simulink model "Encoding_Unstable_system"  (R2021a)
settings: Solver=VariableStepAuto  StartTime=0.0  StopTime=100  RelTol=1e-3
values from neighbouring files (symbols this model uses):
  sample_time = 1    [main1.m]    (also in main2.m)
undefined symbols (not defined in the file or in its folder): Discrete, Time
libraries: dspsrcs4 x2, ctrlSharedLib x1
settings Model: Creator=mehra  LastModifiedBy=mehra

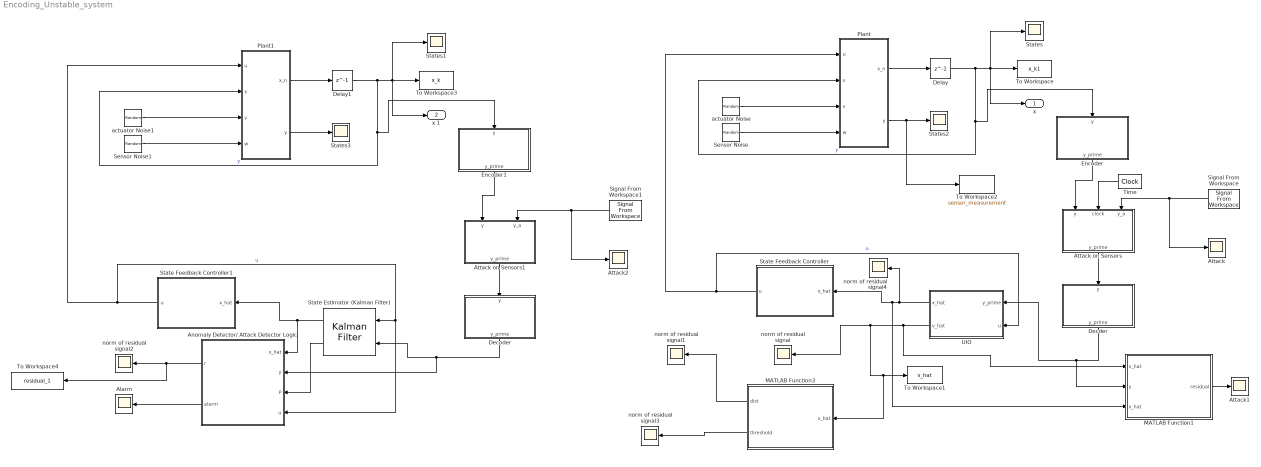
== system Encoding_Unstable_system ==
  Alarm : Scope
  Anomaly Detector/ Attack Detector Logic : MATLAB Function  TreatAsAtomicUnit=on
  Attack : Scope
  Attack on Sensors : MATLAB Function  TreatAsAtomicUnit=on
  Attack on Sensors1 : MATLAB Function  TreatAsAtomicUnit=on
  Attack1 : Scope
  Attack2 : Scope
  Decder : MATLAB Function  TreatAsAtomicUnit=on
  Decoder : MATLAB Function  TreatAsAtomicUnit=on
  Delay : Delay  DelayLength=1  InitialCondition=[0;0]  SampleTime=sample_time
  Delay1 : Delay  DelayLength=1  InitialCondition=[0;0]  SampleTime=sample_time
  Encoder : MATLAB Function  TreatAsAtomicUnit=on
  Encoder1 : MATLAB Function  TreatAsAtomicUnit=on
  MATLAB Function1 : MATLAB Function  TreatAsAtomicUnit=on
  MATLAB Function3 : MATLAB Function  TreatAsAtomicUnit=on
  Plant : MATLAB Function  TreatAsAtomicUnit=on
  Plant1 : MATLAB Function  TreatAsAtomicUnit=on
  Sensor Noise : RandomNumber  Mean=[0 0]  Variance=[0.0001 0.0001]  Seed=[randi(100) randi(100)]  SampleTime=sample_time
  Sensor Noise1 : RandomNumber  Mean=[0 0]  Variance=[0.01 0.01]  Seed=[randi(100) randi(100)]  SampleTime=sample_time
  Signal From Workspace : dspsrcs4/Signal From Workspace  X=y_a  Ts=sample_time  nsamps=1  OutputAfterFinalValue=Cyclic repetition  ignoreOrWarnInputAndFrameLengths=off  OutputFrames=off
  Signal From Workspace1 : dspsrcs4/Signal From Workspace  X=y_a  Ts=sample_time  nsamps=1  OutputAfterFinalValue=Cyclic repetition  ignoreOrWarnInputAndFrameLengths=off  OutputFrames=off
  State Estimator (Kalman Filter) : ctrlSharedLib/Kalman Filter  TimeDomain=Discrete-Time  UseCurrentEstimator=on  ModelSource=Individual A, B, C, D matrices  ModelSourceVariable=ss(0.95,1,1,0,1)  A=[0.8 0; 0.5 1]  B=[1;0.5]  C=[2 0.5;0 1]  D=0  NumberOfStates=1  NumberOfInputs=1  NumberOfOutputs=1  InitialEstimateSource=Dialog  X0=[0 0]'  P0=10  UseK=off  UseGH=off  NumberOfProcessNoiseInputs=1  G=1  TimeInvariantG=on  H=0  TimeInvariantH=on  Q=0.001  TimeInvariantQ=on  R=0.001  TimeInvariantR=on  N=0  TimeInvariantN=on  AddInputPort=on  AddEnablePort=off  OutputEstimatedY=off  OutputP=on  Ts=sample_time
  State Feedback Controller : MATLAB Function  TreatAsAtomicUnit=on
  State Feedback Controller1 : MATLAB Function  TreatAsAtomicUnit=on
  States{,1..3} (4 alike) : Scope
  Time : DigitalClock  SampleTime=sample_time
  To Workspace : ToWorkspace  VariableName=x_k1  SaveFormat=Timeseries  SampleTime=sample_time
  To Workspace1 : ToWorkspace  VariableName=v_hat  SaveFormat=Timeseries  SampleTime=sample_time
  To Workspace2 : ToWorkspace  VariableName=sensor_measurement  SaveFormat=Timeseries  SampleTime=sample_time
  To Workspace3 : ToWorkspace  VariableName=x_k  SaveFormat=Timeseries  SampleTime=sample_time
  To Workspace4 : ToWorkspace  VariableName=residual_1  SaveFormat=Timeseries  SampleTime=sample_time
  UIO : Subsystem
  actuator Noise : RandomNumber  Mean=[0 0]  Variance=[0.0001 0.0001]  Seed=[randi(100) randi(100)]  SampleTime=sample_time
  actuator Noise1 : RandomNumber  Mean=[0 0]  Variance=[0.0001 0.0001]  Seed=[randi(100) randi(100)]  SampleTime=sample_time
  norm of residual signal{,1..4} (5 alike) : Scope
  "x " : Outport  VectorParamsAs1DForOutWhenUnconnected=off
  x 1 : Outport  Port=2  VectorParamsAs1DForOutWhenUnconnected=off
  wires:
  Time/1 -> Attack on Sensors/2(clock)
  Signal From Workspace/1 -> Attack/1, Attack on Sensors/3(y_a)
  Encoder/1(y_prime) -> Attack on Sensors/1(y)
  Plant/2(y) -> To Workspace2/1, States2/1
  Decder/1(y_prime) -> MATLAB Function1/2(y), UIO/1(y_prime)
  actuator Noise/1 -> Plant/3(v)
  State Feedback Controller/1(u) -> UIO/2(u), Plant/1(u)  "u"
  Delay/1 -> "x "/1, States/1, To Workspace/1, Plant/2(x), Encoder/1(y)  "y"
  Attack on Sensors/1(y_prime) -> Decder/1(y)
  Sensor Noise/1 -> Plant/4(w)
  Plant/1(x_n) -> Delay/1
  UIO/1(x_hat) -> norm of residual signal4/1, MATLAB Function1/3(x_hat), State Feedback Controller/1(x_hat)
  UIO/2(v_hat) -> MATLAB Function1/1(v_hat), MATLAB Function3/1(v_hat), To Workspace1/1, norm of residual signal/1
  MATLAB Function3/1(dist) -> norm of residual signal1/1
  MATLAB Function3/2(threshold) -> norm of residual signal3/1
  MATLAB Function1/1(residual) -> Attack1/1
  State Estimator (Kalman Filter)/2 -> Anomaly Detector/ Attack Detector Logic/3(P)
  State Feedback Controller1/1(u) -> State Estimator (Kalman Filter)/1, Anomaly Detector/ Attack Detector Logic/4(u), Plant1/1(u)  "u"
  Anomaly Detector/ Attack Detector Logic/2(alarm) -> Alarm/1
  actuator Noise1/1 -> Plant1/3(v)
  Decoder/1(y_prime) -> Anomaly Detector/ Attack Detector Logic/2(y), State Estimator (Kalman Filter)/2
  Signal From Workspace1/1 -> Attack2/1, Attack on Sensors1/2(y_a)
  Anomaly Detector/ Attack Detector Logic/1(r) -> To Workspace4/1, norm of residual signal2/1
  Attack on Sensors1/1(y_prime) -> Decoder/1(y)
  Encoder1/1(y_prime) -> Attack on Sensors1/1(y)
  Delay1/1 -> x 1/1, States1/1, To Workspace3/1, Plant1/2(x), Encoder1/1(y)  "y"
  Plant1/2(y) -> States3/1
  State Estimator (Kalman Filter)/1 -> Anomaly Detector/ Attack Detector Logic/1(x_hat), State Feedback Controller1/1(x_hat)
  Sensor Noise1/1 -> Plant1/4(w)
  Plant1/1(x_n) -> Delay1/1

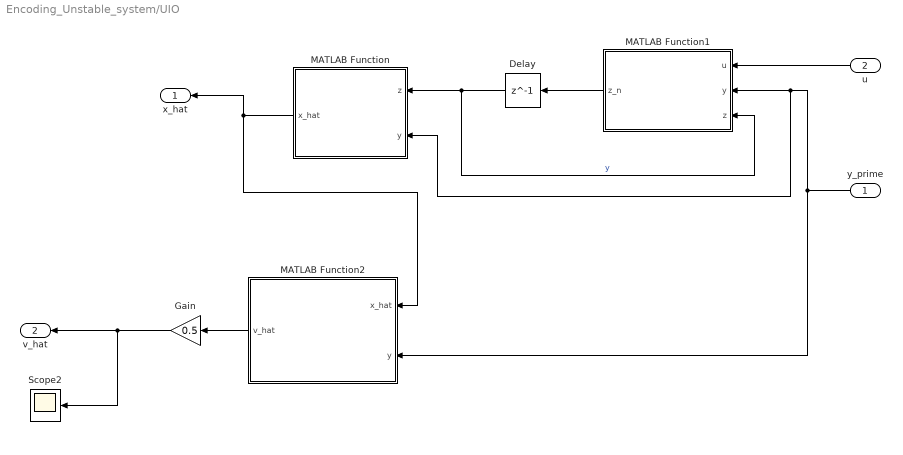
== system Encoding_Unstable_system/UIO ==
  y_prime : Inport
  u : Inport  Port=2
  Delay : Delay  DelayLength=1  InitialCondition=zeros(2,1)
  Gain : Gain  Gain=0.5
  MATLAB Function : MATLAB Function  TreatAsAtomicUnit=on
  MATLAB Function1 : MATLAB Function  TreatAsAtomicUnit=on
  MATLAB Function2 : MATLAB Function  TreatAsAtomicUnit=on
  Scope2 : Scope
  x_hat : Outport  VectorParamsAs1DForOutWhenUnconnected=off
  v_hat : Outport  Port=2  VectorParamsAs1DForOutWhenUnconnected=off
  wires:
  MATLAB Function1/1(z_n) -> Delay/1
  u/1 -> MATLAB Function1/1(u)
  y_prime/1 -> MATLAB Function/2(y), MATLAB Function1/2(y), MATLAB Function2/2(y)
  Delay/1 -> MATLAB Function1/3(z), MATLAB Function/1(z)  "y"
  MATLAB Function/1(x_hat) -> x_hat/1, MATLAB Function2/1(x_hat)
  MATLAB Function2/1(v_hat) -> Gain/1
  Gain/1 -> Scope2/1, v_hat/1

== matlab function Encoding_Unstable_system/Anomaly Detector// Attack Detector Logic ==
  data: x_hat input; y input; r output; P input; alarm output; u input
function [r, alarm] = Detector(x_hat,y, P, u)
% this function should contain the detection strategy

% for the chi square detector "P" should be the name of detection signal and
% "tau" the name of threshold
A = [0.8 0; 0.5 1];
B = [1;0.5];
C = [2 0.5;0 1];
threshold = chi2inv(0.99,2);
sigma = ((C)*(P)*(C')) + 0.01;
r = 0.8*norm(y' - C*(A*x_hat + B*u),2);
z = (r') * (inv(sigma)) * r;
if z<=threshold
    alarm = 0;
else
    alarm = 1;
end
alarm = alarm;
residual = z;
threshold = threshold;
end

== matlab function Encoding_Unstable_system/Attack on Sensors1 ==
  data: y input; y_prime output; y_a input
function y_prime = fcn(y, y_a)
% this function should contain the attacker action on the sensor
% measurements
sigma1 = [2 -0.5;-0.5 1];
sigma2 = [1 -1;2 0];

y_prime = y_a;
% y_prime = y;

end

== matlab function Encoding_Unstable_system/Decoder ==
  data: y input; y_prime output
function y_prime = fcn(y)
% this function should contain the attacker action on the sensor
% measurements
sigma1 = [2 -0.5;-0.5 1];
sigma2 = [1 -1;2 0];
% y_prime = y*inv(sigma1);
y_prime = y;
end

== matlab function Encoding_Unstable_system/Encoder1 ==
  data: y input; y_prime output
function y_prime = fcn(y)
% this function should contain the attacker action on the sensor
% measurements
sigma1 = [2 -0.5;-0.5 1];
sigma2 = [1 -1;2 0];
% y_prime = y'*sigma1;
y_prime = y;
end

== matlab function Encoding_Unstable_system/Plant1 ==
  data: x_n output; u input; y output; x input; v input; w input
function [x_n, y] = fcn(u, x, v, w)

%A=[1.0000    0.0001   -0.0010;0.5747    1.0000   -0.0003;0.0162    0.0000    1.0000];
%B = [0.1   -0.2; -0.0536    0.0332;0.1955   -0.5294];

A = [0.8 0; 0.5 1];
B = [1;0.5];
C = [2 0.5;0 1];
D = 0;

x_n = A*x + B*u + v;
y = C*x + D*u + w;

== matlab function Encoding_Unstable_system/State Feedback Controller1 ==
  data: x_hat input; u output
function u  = Controller(x_hat)
%two tanks model 



K = [-1  -4];

u = K*x_hat;

== matlab function Encoding_Unstable_system/Plant ==
  data: x_n output; u input; y output; x input; v input; w input
function [x_n, y] = fcn(u, x, v, w)

%A=[1.0000    0.0001   -0.0010;0.5747    1.0000   -0.0003;0.0162    0.0000    1.0000];
%B = [0.1   -0.2; -0.0536    0.0332;0.1955   -0.5294];

A = [0.8 0; 0.5 1];
B = [1;0.5];
C = [2 0.5;0 1];
D = 0;

x_n = A*x + B*u + v;
y = C*x + D*u + w;

== matlab function Encoding_Unstable_system/Attack on Sensors ==
  data: y input; y_prime output; clock input; y_a input
function y_prime = fcn(y, clock, y_a)
% this function should contain the attacker action on the sensor
% measurements
sigma1 = [2 -0.5;-0.5 1];
sigma2 = [1 -1;2 0];

% y_prime = y_a;
y_prime = y;

end

== matlab function Encoding_Unstable_system/State Feedback Controller ==
  data: x_hat input; u output
function u  = Controller(x_hat)
%two tanks model 



K = [0.1 -0.1];

u = K*x_hat;

== matlab function Encoding_Unstable_system/MATLAB Function3 ==
  data: v_hat input; dist output; threshold output
function [dist,threshold] = Anomaly_Detector(v_hat)


sigma = 0.0136;
mu = 0;
% a = 0.0150;
% b = sqrt(2*pi);
% c = 1/(a.*b);
c = sqrt(sigma) * sqrt(2*pi)
% dist = (1./c) *(exp(-0.5*(1/sigma)*(v_hat - mu)^2))*1/29.5893;
dist = abs(log2(1/(2*pi*sigma)*exp(-(v_hat-mu).^2/(2*sigma^2)))/2.5);


% pd = makedist('Normal','mu',mu,'sigma',sigma);
% dist = pdf(pd,v_hat)
threshold = 0.9;

if dist<threshold
    alarm = 1;
%     prob = 0;
% abs(v_hat) <= 0.13
else
    alarm = 0;
%     prob = 1;



end

== matlab function Encoding_Unstable_system/Encoder ==
  data: y input; y_prime output
function y_prime = fcn(y)
% this function should contain the attacker action on the sensor
% measurements

trans = [-0.547381274157748,0.836883349518582;0.836883349518582,0.547381274157748];

y_prime = y'*trans;
% y_prime = y;
end

== matlab function Encoding_Unstable_system/Decder ==
  data: y input; y_prime output
function y_prime = fcn(y)
% this function should contain the attacker action on the sensor
% measurements
trans = [-0.547381274157748,0.836883349518582;0.836883349518582,0.547381274157748];

y_prime = y*trans';
% y_prime = y;
end

== matlab function Encoding_Unstable_system/UIO/MATLAB Function ==
  data: z input; x_hat output; y input
function x_hat = estimator(z,y)

M = [0.666666666666667,-0.666666666666667;
    0.666666666666667,-0.666666666666667];

x_hat = z + M*y';

== matlab function Encoding_Unstable_system/UIO/MATLAB Function1 ==
  data: u input; z_n output; y input; z input
function z_n = UIO(u,y,z)

A = [0.8 0; 0.5 1];
B = [1;0.5];
C = [2 0.5;0 1];
D = 0;

M = [0.666666666666667,-0.666666666666667;
    0.666666666666667,-0.666666666666667];




L6 = [-0.0515    0.3474;
   -0.2058    1.3897];

z_n = (eye(2)-M*C)*(A*z + A*M*y'+B*u) + L6*(y' - C*z - C*M*y');

x_hat = z + M*y';

== matlab function Encoding_Unstable_system/UIO/MATLAB Function2 ==
  data: x_hat input; v_hat output; y input
function v_hat = unknown_estimator(x_hat,y)

A = [0.8 0; 0.5 1];
B = [1;0.5];
C = [2 0.5;0 1];
% D = 0;

E = [1;1];
D = [1;1];

v_hat = pinv(D)*y' - pinv(D)*C*x_hat;

== matlab function Encoding_Unstable_system/MATLAB Function1 ==
  data: v_hat input; residual output; y input; x_hat input
function residual = Anomaly_Detector(v_hat,y,x_hat)


A = [0.8 0; 0.5 1];
B = [1;0.5];
C = [2 0.5;0 1];

residual = y' - C*x_hat - v_hat

end
